simulink model "simulator"  (R2024b)
settings: Solver=ode4  StartTime=0.0  StopTime=inf  RelTol=1e-3
values from neighbouring files (symbols this model uses):
  list24 = [0,1,2,3,4,5,6,7,8,9,10,11,12,13,14,15,16,17,18,19,20,21,22,23]*3600    [init.m]
  qOut_median = 30/3600    (= 0.00833333333333)    [init.m]
  qV_max = 120/3600    (= 0.0333333333333)    [init.m]
libraries: simulink x2
settings Model: PacingRate=1000  Creator=antho  LastModifiedBy=antho

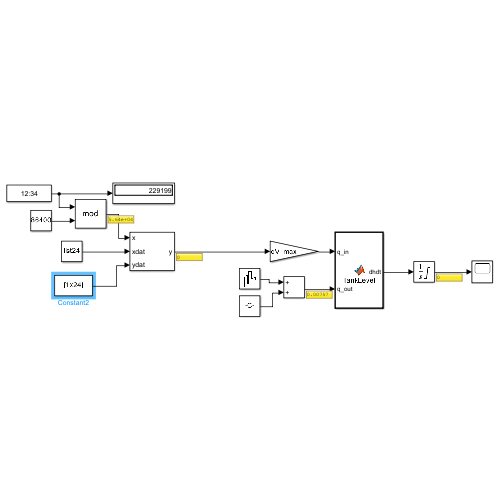
[thumbnail: Simulink's stored preview of the top-level diagram]
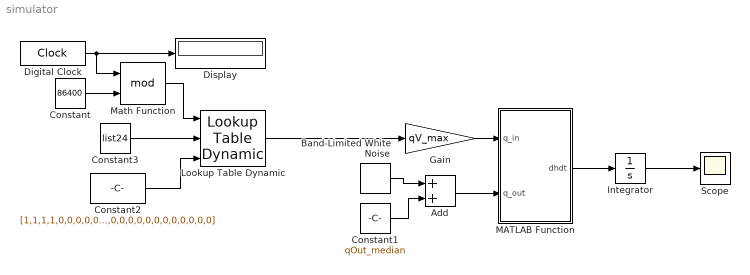
== system simulator ==
  Add : Sum
  Band-Limited White Noise : simulink/Sources/Band-Limited White Noise  Cov=[0.00001]  Ts=1  seed=[23341]
  Constant : Constant  Value=86400
  Constant1 : Constant  Value=qOut_median
  Constant2 : Constant  Value=[1,1,1,1,0,0,0,0,0,0,0,0,0,0,0,0,0,0,0,0,0,0,0,0]
  Constant3 : Constant  Value=list24
  Digital Clock : DigitalClock
  Display : Display
  Gain : Gain  Gain=qV_max
  Integrator : Integrator  LimitOutput=on  UpperSaturationLimit=2  LowerSaturationLimit=0
  Lookup Table Dynamic : simulink/Lookup Tables/Lookup Table Dynamic  LookUpMeth=Interpolation-Use End Values  OutDataType=fixdt('double')  OutScaling=2^-10  OutputDataTypeScalingMode=Specify via dialog  OutDataTypeStr=double  DoSatur=off
  MATLAB Function : MATLAB Function  TreatAsAtomicUnit=on
  Math Function : Math  Operator=mod
  Scope : Scope
  wires:
  MATLAB Function/1(dhdt) -> Integrator/1
  Gain/1 -> MATLAB Function/1(q_in)
  Integrator/1 -> Scope/1
  Band-Limited White Noise/1 -> Add/1
  Constant1/1 -> Add/2
  Add/1 -> MATLAB Function/2(q_out)
  Constant2/1 -> Lookup Table Dynamic/3
  Digital Clock/1 -> Display/1, Math Function/1
  Lookup Table Dynamic/1 -> Gain/1
  Constant3/1 -> Lookup Table Dynamic/2
  Math Function/1 -> Lookup Table Dynamic/1
  Constant/1 -> Math Function/2

== matlab function simulator/MATLAB Function ==
  data: dhdt output; q_in input; q_out input; A parameter
function dhdt = TankLevel(q_in,q_out, A)

dhdt = (1/A)*(q_in-q_out);
